simulink model "first_design"  (R2022a)
settings: Solver=VariableStepAuto  StartTime=0.0  StopTime=10.0  RelTol=1e-3
undefined symbols (not defined in the file or in its folder): dfm_m1, dfm_m2, dfm_sm, dfm_up, dgsm0, dgup0, dsm_m1, dsm_m2, dsm_sm, dsm_up, dsp_m1, dsp_m2, dsp_sm, dsp_up, dup_m1, dup_m2, dup_sm, dup_up, gfm_m1, gfm_m2, gfm_sm, gfm_up, gsm0, gsm_sm, gsm_up, gsp_m1, gsp_m2, gsp_sm, gsp_up, gup0, gup_sm, gup_up
libraries: simulink x4
settings Model: Creator=chris  LastModifiedBy=chris

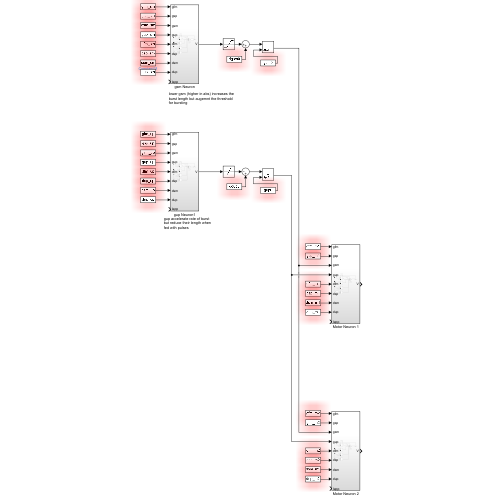
[thumbnail: Simulink's stored preview of the top-level diagram]
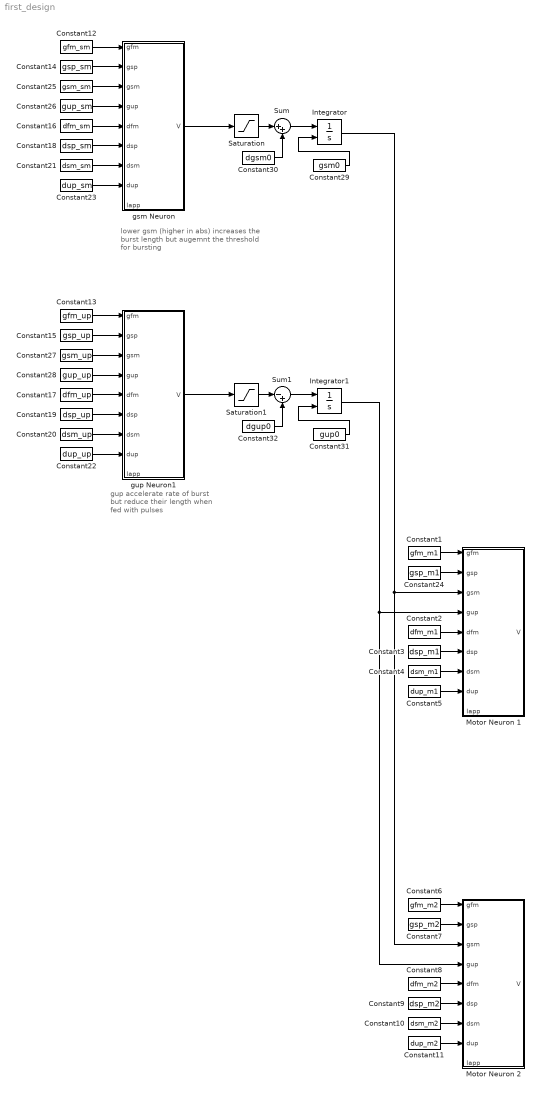
== system first_design ==
  note: lower gsm (higher in abs) increases the
      | burst length but augemnt the threshold
      | for bursting
  note: gup accelerate rate of burst
      | but reduce their length when
      | fed with pulses
  Constant1 : Constant  Value=gfm_m1
  Constant10 : Constant  Value=dsm_m2
  Constant11 : Constant  Value=dup_m2
  Constant12 : Constant  Value=gfm_sm
  Constant13 : Constant  Value=gfm_up
  Constant14 : Constant  Value=gsp_sm
  Constant15 : Constant  Value=gsp_up
  Constant16 : Constant  Value=dfm_sm
  Constant17 : Constant  Value=dfm_up
  Constant18 : Constant  Value=dsp_sm
  Constant19 : Constant  Value=dsp_up
  Constant2 : Constant  Value=dfm_m1
  Constant20 : Constant  Value=dsm_up
  Constant21 : Constant  Value=dsm_sm
  Constant22 : Constant  Value=dup_up
  Constant23 : Constant  Value=dup_sm
  Constant24 : Constant  Value=gsp_m1
  Constant25 : Constant  Value=gsm_sm
  Constant26 : Constant  Value=gup_sm
  Constant27 : Constant  Value=gsm_up
  Constant28 : Constant  Value=gup_up
  Constant29 : Constant  Value=gsm0
  Constant3 : Constant  Value=dsp_m1
  Constant30 : Constant  Value=dgsm0
  Constant31 : Constant  Value=gup0
  Constant32 : Constant  Value=dgup0
  Constant4 : Constant  Value=dsm_m1
  Constant5 : Constant  Value=dup_m1
  Constant6 : Constant  Value=gfm_m2
  Constant7 : Constant  Value=gsp_m2
  Constant8 : Constant  Value=dfm_m2
  Constant9 : Constant  Value=dsp_m2
  Integrator : Integrator  InitialConditionSource=external  InitialCondition=gsm0
  Integrator1 : Integrator  InitialConditionSource=external  InitialCondition=gsm0
  Motor Neuron 1 : Subsystem
  Motor Neuron 2 : Subsystem
  Saturation : Saturate  UpperLimit=5  LowerLimit=0
  Saturation1 : Saturate  UpperLimit=5  LowerLimit=0
  Sum : Sum  Inputs=|++
  Sum1 : Sum  Inputs=|-+
  gsm Neuron : Subsystem
  gup Neuron1 : Subsystem
  wires:
  Constant24/1 -> Motor Neuron 1/2(gsp)
  Constant1/1 -> Motor Neuron 1/1(gfm)
  Constant2/1 -> Motor Neuron 1/5(dfm)
  Constant3/1 -> Motor Neuron 1/6(dsp)
  Constant4/1 -> Motor Neuron 1/7(dsm)
  Constant5/1 -> Motor Neuron 1/8(dup)
  Constant6/1 -> Motor Neuron 2/1(gfm)
  Constant7/1 -> Motor Neuron 2/2(gsp)
  Constant8/1 -> Motor Neuron 2/5(dfm)
  Constant9/1 -> Motor Neuron 2/6(dsp)
  Constant10/1 -> Motor Neuron 2/7(dsm)
  Constant11/1 -> Motor Neuron 2/8(dup)
  Constant12/1 -> gsm Neuron/1(gfm)
  Constant13/1 -> gup Neuron1/1(gfm)
  Constant14/1 -> gsm Neuron/2(gsp)
  Constant15/1 -> gup Neuron1/2(gsp)
  Constant16/1 -> gsm Neuron/5(dfm)
  Constant17/1 -> gup Neuron1/5(dfm)
  Constant18/1 -> gsm Neuron/6(dsp)
  Constant19/1 -> gup Neuron1/6(dsp)
  Constant20/1 -> gup Neuron1/7(dsm)
  Constant21/1 -> gsm Neuron/7(dsm)
  Constant22/1 -> gup Neuron1/8(dup)
  Constant23/1 -> gsm Neuron/8(dup)
  Constant25/1 -> gsm Neuron/3(gsm)
  Constant26/1 -> gsm Neuron/4(gup)
  Constant27/1 -> gup Neuron1/3(gsm)
  Constant28/1 -> gup Neuron1/4(gup)
  gsm Neuron/1(V) -> Saturation/1
  Constant29/1 -> Integrator/2
  Saturation/1 -> Sum/1
  Sum/1 -> Integrator/1
  Constant30/1 -> Sum/2
  Sum1/1 -> Integrator1/1
  Constant32/1 -> Sum1/2
  Saturation1/1 -> Sum1/1
  Constant31/1 -> Integrator1/2
  gup Neuron1/1(V) -> Saturation1/1
  Integrator1/1 -> Motor Neuron 2/4(gup), Motor Neuron 1/4(gup)
  Integrator/1 -> Motor Neuron 2/3(gsm), Motor Neuron 1/3(gsm)

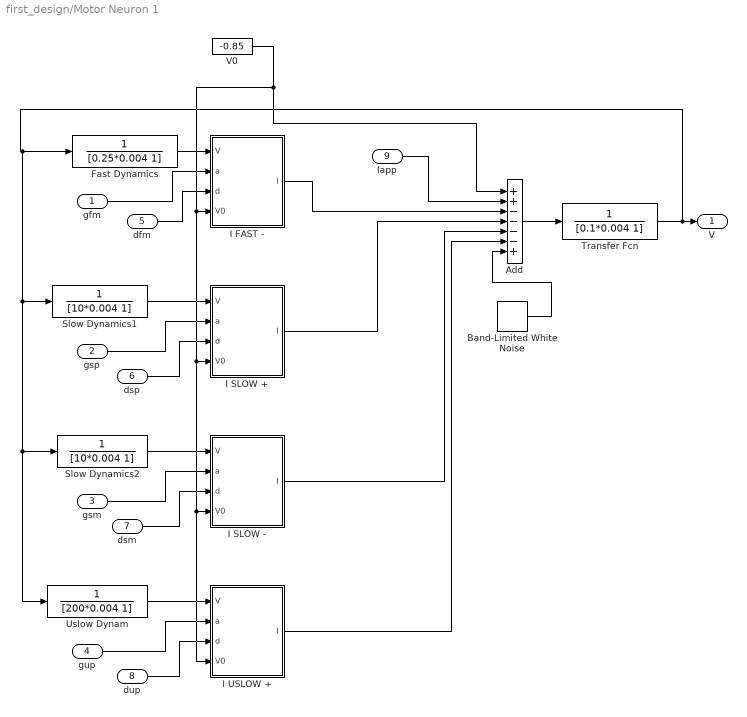
== system first_design/Motor Neuron 1 ==
  gfm : Inport
  gsp : Inport  Port=2
  gsm : Inport  Port=3
  gup : Inport  Port=4
  dfm : Inport  Port=5
  dsp : Inport  Port=6
  dsm : Inport  Port=7
  dup : Inport  Port=8
  Iapp : Inport  Port=9
  Add : Sum  Inputs=++----+
  Band-Limited White Noise : simulink/Sources/Band-Limited White Noise  Cov=[0.00000]  Ts=0.001  seed=[23341]
  Fast Dynamics : TransferFcn  Denominator=[0.25*0.004 1]
  I FAST - : MATLAB Function  TreatAsAtomicUnit=on
  I SLOW + : MATLAB Function  TreatAsAtomicUnit=on
  I SLOW - : MATLAB Function  TreatAsAtomicUnit=on
  I USLOW + : MATLAB Function  TreatAsAtomicUnit=on
  Slow Dynamics1 : TransferFcn  Denominator=[10*0.004 1]
  Slow Dynamics2 : TransferFcn  Denominator=[10*0.004 1]
  Transfer Fcn : TransferFcn  Denominator=[0.1*0.004 1]
  Uslow Dynam : TransferFcn  Denominator=[200*0.004 1]
  V0 : Constant  Value=-0.85
  V : Outport
  wires:
  dup/1 -> I USLOW +/3(d)
  gsm/1 -> I SLOW -/2(a)
  dsm/1 -> I SLOW -/3(d)
  gup/1 -> I USLOW +/2(a)
  Iapp/1 -> Add/2
  Uslow Dynam/1 -> I USLOW +/1(V)
  Add/1 -> Transfer Fcn/1
  Slow Dynamics1/1 -> I SLOW +/1(V)
  Slow Dynamics2/1 -> I SLOW -/1(V)
  I FAST -/1(I) -> Add/3
  I USLOW +/1(I) -> Add/6
  V0/1 -> I USLOW +/4(V0), I SLOW -/4(V0), I SLOW +/4(V0), I FAST -/4(V0), Add/1
  dsp/1 -> I SLOW +/3(d)
  gsp/1 -> I SLOW +/2(a)
  dfm/1 -> I FAST -/3(d)
  gfm/1 -> I FAST -/2(a)
  Fast Dynamics/1 -> I FAST -/1(V)
  I SLOW -/1(I) -> Add/5
  Transfer Fcn/1 -> Uslow Dynam/1, Slow Dynamics2/1, Slow Dynamics1/1, Fast Dynamics/1, V/1
  I SLOW +/1(I) -> Add/4
  Band-Limited White Noise/1 -> Add/7

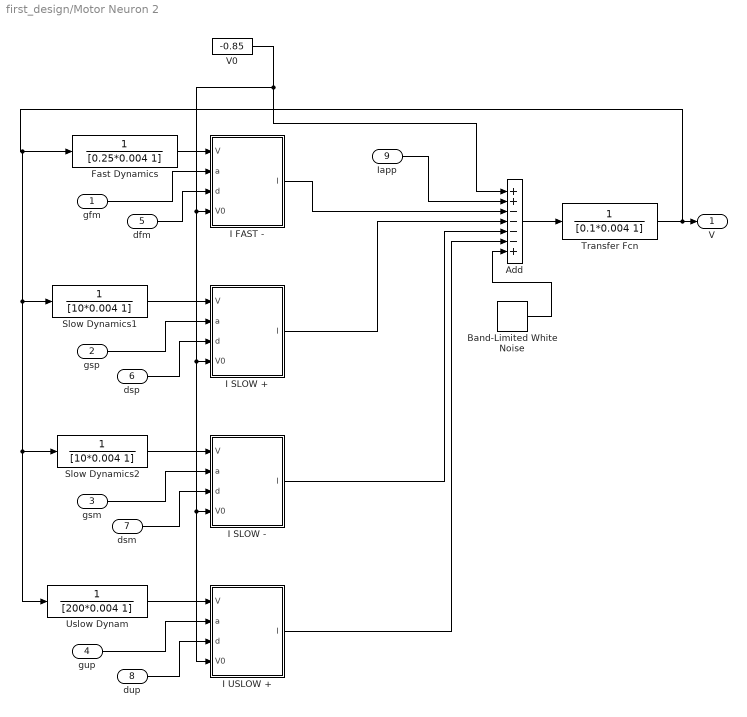
== system first_design/Motor Neuron 2 ==
  gfm : Inport
  gsp : Inport  Port=2
  gsm : Inport  Port=3
  gup : Inport  Port=4
  dfm : Inport  Port=5
  dsp : Inport  Port=6
  dsm : Inport  Port=7
  dup : Inport  Port=8
  Iapp : Inport  Port=9
  Add : Sum  Inputs=++----+
  Band-Limited White Noise : simulink/Sources/Band-Limited White Noise  Cov=[0.00000]  Ts=0.001  seed=[23341]
  Fast Dynamics : TransferFcn  Denominator=[0.25*0.004 1]
  I FAST - : MATLAB Function  TreatAsAtomicUnit=on
  I SLOW + : MATLAB Function  TreatAsAtomicUnit=on
  I SLOW - : MATLAB Function  TreatAsAtomicUnit=on
  I USLOW + : MATLAB Function  TreatAsAtomicUnit=on
  Slow Dynamics1 : TransferFcn  Denominator=[10*0.004 1]
  Slow Dynamics2 : TransferFcn  Denominator=[10*0.004 1]
  Transfer Fcn : TransferFcn  Denominator=[0.1*0.004 1]
  Uslow Dynam : TransferFcn  Denominator=[200*0.004 1]
  V0 : Constant  Value=-0.85
  V : Outport
  wires:
  dup/1 -> I USLOW +/3(d)
  gsm/1 -> I SLOW -/2(a)
  dsm/1 -> I SLOW -/3(d)
  gup/1 -> I USLOW +/2(a)
  Iapp/1 -> Add/2
  Uslow Dynam/1 -> I USLOW +/1(V)
  Add/1 -> Transfer Fcn/1
  Slow Dynamics1/1 -> I SLOW +/1(V)
  Slow Dynamics2/1 -> I SLOW -/1(V)
  I FAST -/1(I) -> Add/3
  I USLOW +/1(I) -> Add/6
  V0/1 -> I USLOW +/4(V0), I SLOW -/4(V0), I SLOW +/4(V0), I FAST -/4(V0), Add/1
  dsp/1 -> I SLOW +/3(d)
  gsp/1 -> I SLOW +/2(a)
  dfm/1 -> I FAST -/3(d)
  gfm/1 -> I FAST -/2(a)
  Fast Dynamics/1 -> I FAST -/1(V)
  I SLOW -/1(I) -> Add/5
  Transfer Fcn/1 -> Uslow Dynam/1, Slow Dynamics2/1, Slow Dynamics1/1, Fast Dynamics/1, V/1
  I SLOW +/1(I) -> Add/4
  Band-Limited White Noise/1 -> Add/7

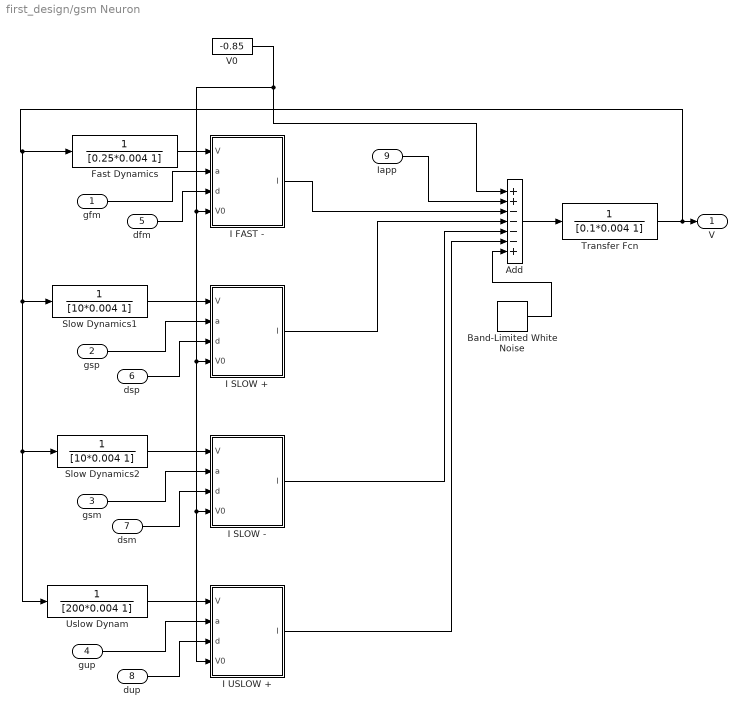
== system first_design/gsm Neuron ==
  gfm : Inport
  gsp : Inport  Port=2
  gsm : Inport  Port=3
  gup : Inport  Port=4
  dfm : Inport  Port=5
  dsp : Inport  Port=6
  dsm : Inport  Port=7
  dup : Inport  Port=8
  Iapp : Inport  Port=9
  Add : Sum  Inputs=++----+
  Band-Limited White Noise : simulink/Sources/Band-Limited White Noise  Cov=[0.00000]  Ts=0.001  seed=[23341]
  Fast Dynamics : TransferFcn  Denominator=[0.25*0.004 1]
  I FAST - : MATLAB Function  TreatAsAtomicUnit=on
  I SLOW + : MATLAB Function  TreatAsAtomicUnit=on
  I SLOW - : MATLAB Function  TreatAsAtomicUnit=on
  I USLOW + : MATLAB Function  TreatAsAtomicUnit=on
  Slow Dynamics1 : TransferFcn  Denominator=[10*0.004 1]
  Slow Dynamics2 : TransferFcn  Denominator=[10*0.004 1]
  Transfer Fcn : TransferFcn  Denominator=[0.1*0.004 1]
  Uslow Dynam : TransferFcn  Denominator=[200*0.004 1]
  V0 : Constant  Value=-0.85
  V : Outport
  wires:
  dup/1 -> I USLOW +/3(d)
  gsm/1 -> I SLOW -/2(a)
  dsm/1 -> I SLOW -/3(d)
  gup/1 -> I USLOW +/2(a)
  Iapp/1 -> Add/2
  Uslow Dynam/1 -> I USLOW +/1(V)
  Add/1 -> Transfer Fcn/1
  Slow Dynamics1/1 -> I SLOW +/1(V)
  Slow Dynamics2/1 -> I SLOW -/1(V)
  I FAST -/1(I) -> Add/3
  I USLOW +/1(I) -> Add/6
  V0/1 -> I USLOW +/4(V0), I SLOW -/4(V0), I SLOW +/4(V0), I FAST -/4(V0), Add/1
  dsp/1 -> I SLOW +/3(d)
  gsp/1 -> I SLOW +/2(a)
  dfm/1 -> I FAST -/3(d)
  gfm/1 -> I FAST -/2(a)
  Fast Dynamics/1 -> I FAST -/1(V)
  I SLOW -/1(I) -> Add/5
  Transfer Fcn/1 -> Uslow Dynam/1, Slow Dynamics2/1, Slow Dynamics1/1, Fast Dynamics/1, V/1
  I SLOW +/1(I) -> Add/4
  Band-Limited White Noise/1 -> Add/7

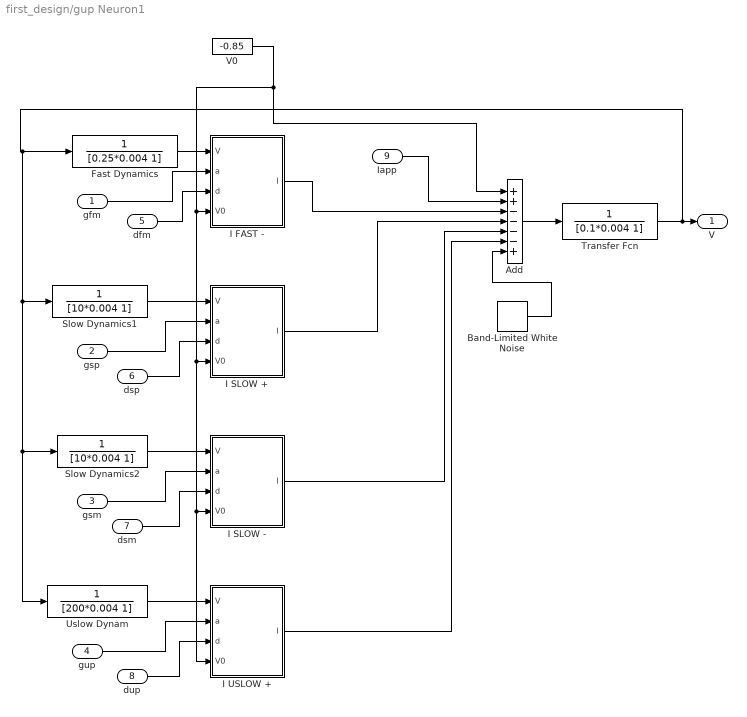
== system first_design/gup Neuron1 ==
  gfm : Inport
  gsp : Inport  Port=2
  gsm : Inport  Port=3
  gup : Inport  Port=4
  dfm : Inport  Port=5
  dsp : Inport  Port=6
  dsm : Inport  Port=7
  dup : Inport  Port=8
  Iapp : Inport  Port=9
  Add : Sum  Inputs=++----+
  Band-Limited White Noise : simulink/Sources/Band-Limited White Noise  Cov=[0.00000]  Ts=0.001  seed=[23341]
  Fast Dynamics : TransferFcn  Denominator=[0.25*0.004 1]
  I FAST - : MATLAB Function  TreatAsAtomicUnit=on
  I SLOW + : MATLAB Function  TreatAsAtomicUnit=on
  I SLOW - : MATLAB Function  TreatAsAtomicUnit=on
  I USLOW + : MATLAB Function  TreatAsAtomicUnit=on
  Slow Dynamics1 : TransferFcn  Denominator=[10*0.004 1]
  Slow Dynamics2 : TransferFcn  Denominator=[10*0.004 1]
  Transfer Fcn : TransferFcn  Denominator=[0.1*0.004 1]
  Uslow Dynam : TransferFcn  Denominator=[200*0.004 1]
  V0 : Constant  Value=-0.85
  V : Outport
  wires:
  dup/1 -> I USLOW +/3(d)
  gsm/1 -> I SLOW -/2(a)
  dsm/1 -> I SLOW -/3(d)
  gup/1 -> I USLOW +/2(a)
  Iapp/1 -> Add/2
  Uslow Dynam/1 -> I USLOW +/1(V)
  Add/1 -> Transfer Fcn/1
  Slow Dynamics1/1 -> I SLOW +/1(V)
  Slow Dynamics2/1 -> I SLOW -/1(V)
  I FAST -/1(I) -> Add/3
  I USLOW +/1(I) -> Add/6
  V0/1 -> I USLOW +/4(V0), I SLOW -/4(V0), I SLOW +/4(V0), I FAST -/4(V0), Add/1
  dsp/1 -> I SLOW +/3(d)
  gsp/1 -> I SLOW +/2(a)
  dfm/1 -> I FAST -/3(d)
  gfm/1 -> I FAST -/2(a)
  Fast Dynamics/1 -> I FAST -/1(V)
  I SLOW -/1(I) -> Add/5
  Transfer Fcn/1 -> Uslow Dynam/1, Slow Dynamics2/1, Slow Dynamics1/1, Fast Dynamics/1, V/1
  I SLOW +/1(I) -> Add/4
  Band-Limited White Noise/1 -> Add/7

== matlab function first_design/Motor Neuron 2/I FAST - ==
  data: V input; I output; a input; d input; V0 input
function I = fcn(V,a,d,V0)

I = a*(tanh(V-d)-tanh(V0-d));

== matlab function first_design/gup Neuron1/I SLOW + ==
  data: V input; I output; a input; d input; V0 input
function I = fcn(V,a,d,V0)

I = a*(tanh(V-d)-tanh(V0-d));

== matlab function first_design/gup Neuron1/I SLOW - ==
  data: V input; I output; a input; d input; V0 input
function I = fcn(V,a,d,V0)

I = a*(tanh(V-d)-tanh(V0-d));

== matlab function first_design/gup Neuron1/I USLOW + ==
  data: V input; I output; a input; d input; V0 input
function I = fcn(V,a,d,V0)

I = a*(tanh(V-d)-tanh(V0-d));

== matlab function first_design/Motor Neuron 1/I FAST - ==
  data: V input; I output; a input; d input; V0 input
function I = fcn(V,a,d,V0)

I = a*(tanh(V-d)-tanh(V0-d));

== matlab function first_design/Motor Neuron 1/I SLOW + ==
  data: V input; I output; a input; d input; V0 input
function I = fcn(V,a,d,V0)

I = a*(tanh(V-d)-tanh(V0-d));

== matlab function first_design/Motor Neuron 1/I SLOW - ==
  data: V input; I output; a input; d input; V0 input
function I = fcn(V,a,d,V0)

I = a*(tanh(V-d)-tanh(V0-d));

== matlab function first_design/Motor Neuron 1/I USLOW + ==
  data: V input; I output; a input; d input; V0 input
function I = fcn(V,a,d,V0)

I = a*(tanh(V-d)-tanh(V0-d));

== matlab function first_design/Motor Neuron 2/I SLOW + ==
  data: V input; I output; a input; d input; V0 input
function I = fcn(V,a,d,V0)

I = a*(tanh(V-d)-tanh(V0-d));

== matlab function first_design/Motor Neuron 2/I SLOW - ==
  data: V input; I output; a input; d input; V0 input
function I = fcn(V,a,d,V0)

I = a*(tanh(V-d)-tanh(V0-d));

== matlab function first_design/Motor Neuron 2/I USLOW + ==
  data: V input; I output; a input; d input; V0 input
function I = fcn(V,a,d,V0)

I = a*(tanh(V-d)-tanh(V0-d));

== matlab function first_design/gsm Neuron/I FAST - ==
  data: V input; I output; a input; d input; V0 input
function I = fcn(V,a,d,V0)

I = a*(tanh(V-d)-tanh(V0-d));

== matlab function first_design/gsm Neuron/I SLOW + ==
  data: V input; I output; a input; d input; V0 input
function I = fcn(V,a,d,V0)

I = a*(tanh(V-d)-tanh(V0-d));

== matlab function first_design/gsm Neuron/I SLOW - ==
  data: V input; I output; a input; d input; V0 input
function I = fcn(V,a,d,V0)

I = a*(tanh(V-d)-tanh(V0-d));

== matlab function first_design/gsm Neuron/I USLOW + ==
  data: V input; I output; a input; d input; V0 input
function I = fcn(V,a,d,V0)

I = a*(tanh(V-d)-tanh(V0-d));

== matlab function first_design/gup Neuron1/I FAST - ==
  data: V input; I output; a input; d input; V0 input
function I = fcn(V,a,d,V0)

I = a*(tanh(V-d)-tanh(V0-d));
